simulink model "Commande"  (R2020b)
settings: Solver=VariableStepAuto  StartTime=0.0  StopTime=1  RelTol=1e-3
undefined symbols (not defined in the file or in its folder): FC, FuelCellLoadFcn, gcbh, ln, sps_rtmsupport, Ts
libraries: simulink x43, powerlib x37, powerlib_meascontrol x7, fuzblock x4, powerlib_extras x2
(part 2 of 3)

== system Commande/INC 1/Fuel Cell Stack/Model/Discrete//Detailed ==
  note: Break Algebraic
      | loop
  Current : Inport
  Op Temp : Inport  Port=2
  H2 : Inport  Port=3
  x_H2 : Inport  Port=4
  Air : Inport  Port=5
  y_O2 : Inport  Port=6
  Pf : Inport  Port=7
  PAir : Inport  Port=8
  Air consumption : Fcn  Expr=60000*FC.Nc*u(1)*FC.R*FC.Tstd/(4*FC.F*FC.Pstd*u(2))
  Bus Creator1 : BusCreator  Inputs=11
  CellVoltage : Subsystem
  Fcn2 : Fcn  Expr=u(1)-FC.Rohm*u(2)
  Fcn3 : Fcn  Expr=FC.Nc*u(1)/(FC.z*FC.F*u(2))*FC.Dh0
  Fuel consumption : Fcn  Expr=60000*FC.Nc*u(1)*FC.R*FC.Tstd/(FC.z*FC.F*FC.Pstd*u(2))
  Gain1 : Gain  Gain=100
  Gain3 : Gain  Gain=100
  Mux{,1,3..4,6} (5 alike) : Mux  Inputs=2
  Product : Product  RndMeth=Zero
  Product1 : Product  Inputs=*/  RndMeth=Zero
  Product2 : Product  RndMeth=Zero
  Saturation1 : Saturate  UpperLimit=0.9999  LowerLimit=0.0001
  Saturation2 : Saturate  UpperLimit=0.9999  LowerLimit=0.0001
  Saturation3 : Saturate  UpperLimit=inf  LowerLimit=1e-6
  Saturation4 : Saturate  UpperLimit=inf  LowerLimit=1e-3
  Saturation6 : Saturate  UpperLimit=inf  LowerLimit=0.001
  Saturation7 : Saturate  UpperLimit=inf  LowerLimit=0.001
  Saturation8 : Saturate  UpperLimit=inf  LowerLimit=200
  Selector : Selector  InputPortWidth=2  IndexOptions=Index vector (dialog)  Indices=[2]  OutputSizes=1
  Unit Delay : UnitDelay  SampleTime=Ts  HasFrameUpgradeWarning=on
  zero avoider : Saturate  UpperLimit=inf  LowerLimit=1e-6  LinearizeAsGain=off
  zero avoider2 : Saturate  UpperLimit=inf  LowerLimit=0  LinearizeAsGain=off
  Voltage : Outport  VectorParamsAs1DForOutWhenUnconnected=off
  m : Outport  Port=2  VectorParamsAs1DForOutWhenUnconnected=off
  wires:
  [E] -> Mux/1
  CellVoltage/7(E) -> [E], Voltage/1
  CellVoltage/5(En) -> Bus Creator1/10  "Nerst voltage En (V)"
  Saturation2/1 -> Mux6/2, CellVoltage/6(y)  "Oxidant composition"
  CellVoltage/4(i0) -> Bus Creator1/9  "Exchange current i0 (A)"
  Product2/1 -> Bus Creator1/6  "Stack consumption (lpm) [Air(Yellow); Fuel(Magenta)]"
  Gain3/1 -> Bus Creator1/3  "Stack Efficiency (%)"
  CellVoltage/1(Fr_AirFuel) -> Bus Creator1/5, Product2/1  "Flow Rate (lpm [Air(Yellow); Fuel(Magenta)]"
  Fuel consumption/1 -> Mux3/2
  Air consumption/1 -> Mux3/1
  Gain1/1 -> Bus Creator1/7  "Utilization (%) [O2(Yellow); H2(Magenta)]"
  Selector/1 -> Mux4/2
  Mux3/1 -> Bus Creator1/4  "Stack consumption (Standard lpm) [Air(Yellow); Fuel(Magenta)]"
  Saturation4/1 -> CellVoltage/5(Air)  "Air flow rate / utilization"
  Saturation3/1 -> CellVoltage/3(H2)  "Fuel flow rate / utilization"
  Bus Creator1/1 -> m/1
  Mux6/1 -> Air consumption/1
  Mux1/1 -> Fuel consumption/1
  CellVoltage/2(Uf_O2H2) -> Product2/2, Gain1/1, Selector/1
  Unit Delay/1 -> Mux6/1, Mux4/1, Mux/2, Bus Creator1/2, Product/2, Mux1/1, CellVoltage/1(i)  "Current"
  Saturation8/1 -> CellVoltage/2(T)  "Operating temperature"
  Saturation7/1 -> CellVoltage/8(PAir)  "Air supply pression"
  Saturation6/1 -> CellVoltage/7(Pf)  "Fuel supply pression"
  Saturation1/1 -> Mux1/2, CellVoltage/4(x)  "Fuel composition"
  Mux4/1 -> Fcn3/1
  PAir/1 -> Saturation7/1
  Pf/1 -> Saturation6/1
  zero avoider2/1 -> Product1/1
  CellVoltage/6(Eoc) -> Bus Creator1/11  "Open circuit voltage Eoc (V)"
  CellVoltage/3(A) -> Bus Creator1/8  "Slope of Tafel curve"
  Air/1 -> Saturation4/1
  Mux/1 -> Fcn2/1
  Fcn2/1 -> Bus Creator1/1, Product/1  "Voltage"
  H2/1 -> Saturation3/1
  x_H2/1 -> Saturation1/1
  y_O2/1 -> Saturation2/1
  Op Temp/1 -> Saturation8/1
  Product/1 -> zero avoider2/1
  Fcn3/1 -> zero avoider/1
  Current/1 -> Unit Delay/1
  Product1/1 -> Gain3/1
  zero avoider/1 -> Product1/2

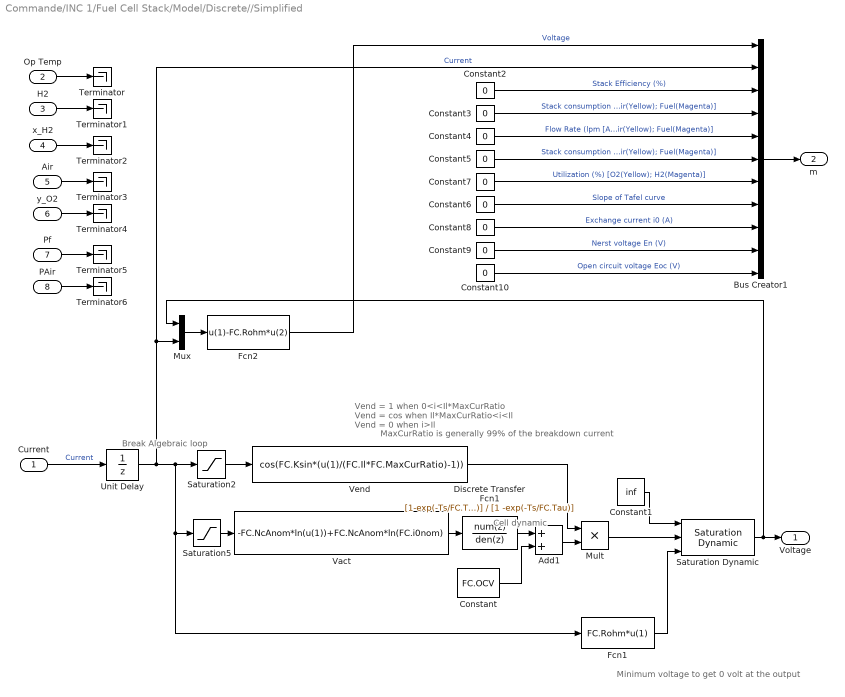
== system Commande/INC 1/Fuel Cell Stack/Model/Discrete//Simplified ==
  note: MaxCurRatio is generally 99% of the breakdown current
  note: Minimum voltage to get 0 volt at the output
  note: Cell dynamic
  note: Vend = 1 when 0<i<Il*MaxCurRatio
      | Vend = cos when Il*MaxCurRatio<i<Il
      | Vend = 0 when i>Il
  note: Break Algebraic
      | loop
  Current : Inport
  Op Temp : Inport  Port=2
  H2 : Inport  Port=3
  x_H2 : Inport  Port=4
  Air : Inport  Port=5
  y_O2 : Inport  Port=6
  Pf : Inport  Port=7
  PAir : Inport  Port=8
  Add1 : Sum
  Bus Creator1 : BusCreator  Inputs=11
  Constant : Constant  Value=FC.OCV
  Constant1 : Constant  Value=inf
  Constant{2..10} (9 alike) : Constant  Value=0
  Discrete Transfer Fcn1 : DiscreteTransferFcn  Numerator=[1-exp(-Ts/FC.Tau)]  Denominator=[1 -exp(-Ts/FC.Tau)]  SampleTime=Ts
  Fcn1 : Fcn  Expr=FC.Rohm*u(1)
  Fcn2 : Fcn  Expr=u(1)-FC.Rohm*u(2)
  Mult : Product
  Mux : Mux  Inputs=2
  Saturation Dynamic : simulink/Discontinuities/Saturation Dynamic  OutMin=[]  OutMax=[]  OutDataTypeStr=Inherit: Same as second input  OutDataType=fixdt(1, 16)  OutScaling=2^-10  DoSatur=off
  Saturation2 : Saturate  UpperLimit=FC.Il  LowerLimit=FC.Il*FC.MaxCurRatio  LinearizeAsGain=off
  Saturation5 : Saturate  UpperLimit=inf  LowerLimit=FC.i0nom  LinearizeAsGain=off
  Terminator{,1..6} (7 alike) : Terminator
  Unit Delay : UnitDelay  SampleTime=Ts  HasFrameUpgradeWarning=on
  Vact : Fcn  Expr=-FC.NcAnom*ln(u(1))+FC.NcAnom*ln(FC.i0nom)
  Vend : Fcn  Expr=cos(FC.Ksin*(u(1)/(FC.Il*FC.MaxCurRatio)-1))
  Voltage : Outport  VectorParamsAs1DForOutWhenUnconnected=off
  m : Outport  Port=2  VectorParamsAs1DForOutWhenUnconnected=off
  wires:
  Fcn2/1 -> Bus Creator1/1  "Voltage"
  Constant9/1 -> Bus Creator1/10  "Nerst voltage En (V)"
  Constant8/1 -> Bus Creator1/9  "Exchange current i0 (A)"
  Constant5/1 -> Bus Creator1/6  "Stack consumption (lpm) [Air(Yellow); Fuel(Magenta)]"
  Constant2/1 -> Bus Creator1/3  "Stack Efficiency (%)"
  Constant4/1 -> Bus Creator1/5  "Flow Rate (lpm [Air(Yellow); Fuel(Magenta)]"
  Constant7/1 -> Bus Creator1/7  "Utilization (%) [O2(Yellow); H2(Magenta)]"
  Constant3/1 -> Bus Creator1/4  "Stack consumption (Standard lpm) [Air(Yellow); Fuel(Magenta)]"
  Bus Creator1/1 -> m/1
  Constant10/1 -> Bus Creator1/11  "Open circuit voltage Eoc (V)"
  Constant6/1 -> Bus Creator1/8  "Slope of Tafel curve"
  PAir/1 -> Terminator6/1
  Pf/1 -> Terminator5/1
  Unit Delay/1 -> Bus Creator1/2, Mux/2, Fcn1/1, Saturation5/1, Saturation2/1  "Current"
  Saturation2/1 -> Vend/1
  Vend/1 -> Mult/1
  Mult/1 -> Saturation Dynamic/2
  Add1/1 -> Mult/2
  Vact/1 -> Discrete Transfer Fcn1/1
  Fcn1/1 -> Saturation Dynamic/3
  Constant1/1 -> Saturation Dynamic/1
  Constant/1 -> Add1/2
  Discrete Transfer Fcn1/1 -> Add1/1
  Saturation Dynamic/1 -> Mux/1, Voltage/1
  y_O2/1 -> Terminator4/1
  Air/1 -> Terminator3/1
  x_H2/1 -> Terminator2/1
  H2/1 -> Terminator1/1
  Op Temp/1 -> Terminator/1
  Current/1 -> Unit Delay/1  "Current"
  Saturation5/1 -> Vact/1
  Mux/1 -> Fcn2/1

== system Commande/P&O/Fuel Cell Stack/Model/Continuous//Detailed ==
  note: Break Algebraic
      | loop
  Current : Inport
  Op Temp : Inport  Port=2
  H2 : Inport  Port=3
  x_H2 : Inport  Port=4
  Air : Inport  Port=5
  y_O2 : Inport  Port=6
  Pf : Inport  Port=7
  PAir : Inport  Port=8
  Air consumption : Fcn  Expr=60000*FC.Nc*u(1)*FC.R*FC.Tstd/(4*FC.F*FC.Pstd*u(2))
  Bus Creator1 : BusCreator  Inputs=11
  CellVoltage : Subsystem
  Constant : Constant  Value=FC.Rohm
  Fcn2 : Fcn  Expr=u(1)-FC.Rohm*u(2)
  Fcn3 : Fcn  Expr=FC.Nc*u(1)/(FC.z*FC.F*u(2))*FC.Dh0
  Fuel consumption : Fcn  Expr=60000*FC.Nc*u(1)*FC.R*FC.Tstd/(FC.z*FC.F*FC.Pstd*u(2))
  Gain1 : Gain  Gain=100
  Gain3 : Gain  Gain=100
  Mux{,1,3..4,6} (5 alike) : Mux  Inputs=2
  Product : Product  RndMeth=Zero
  Product1 : Product  Inputs=*/  RndMeth=Zero
  Product2 : Product  RndMeth=Zero
  Saturation1 : Saturate  UpperLimit=0.9999  LowerLimit=0.0001
  Saturation2 : Saturate  UpperLimit=0.9999  LowerLimit=0.0001
  Saturation3 : Saturate  UpperLimit=inf  LowerLimit=1e-6
  Saturation4 : Saturate  UpperLimit=inf  LowerLimit=1e-3
  Saturation6 : Saturate  UpperLimit=inf  LowerLimit=0.001
  Saturation7 : Saturate  UpperLimit=inf  LowerLimit=0.001
  Saturation8 : Saturate  UpperLimit=inf  LowerLimit=200
  Selector : Selector  InputPortWidth=2  IndexOptions=Index vector (dialog)  Indices=[2]  OutputSizes=1
  Transfer Fcn : TransferFcn  Denominator=[1e-6 1]
  zero avoider : Saturate  UpperLimit=inf  LowerLimit=1e-6  LinearizeAsGain=off
  zero avoider2 : Saturate  UpperLimit=inf  LowerLimit=0  LinearizeAsGain=off
  Voltage : Outport  VectorParamsAs1DForOutWhenUnconnected=off
  m : Outport  Port=2  VectorParamsAs1DForOutWhenUnconnected=off
  wires:
  [E] -> Mux/1
  CellVoltage/7(E) -> Voltage/1, [E]
  CellVoltage/5(En) -> Bus Creator1/10  "Nerst voltage En (V)"
  Saturation2/1 -> Mux6/2, CellVoltage/6(y)  "Oxidant composition"
  CellVoltage/4(i0) -> Bus Creator1/9  "Exchange current i0 (A)"
  Product2/1 -> Bus Creator1/6  "Stack consumption (lpm) [Air(Yellow); Fuel(Magenta)]"
  Gain3/1 -> Bus Creator1/3  "Stack Efficiency (%)"
  CellVoltage/1(Fr_AirFuel) -> Bus Creator1/5, Product2/1  "Flow Rate (lpm [Air(Yellow); Fuel(Magenta)]"
  Fuel consumption/1 -> Mux3/2
  Air consumption/1 -> Mux3/1
  Gain1/1 -> Bus Creator1/7  "Utilization (%) [O2(Yellow); H2(Magenta)]"
  Selector/1 -> Mux4/2
  Mux3/1 -> Bus Creator1/4  "Stack consumption (Standard lpm) [Air(Yellow); Fuel(Magenta)]"
  Saturation4/1 -> CellVoltage/5(Air)  "Air flow rate / utilization"
  Saturation3/1 -> CellVoltage/3(H2)  "Fuel flow rate / utilization"
  Bus Creator1/1 -> m/1
  Mux6/1 -> Air consumption/1
  Mux1/1 -> Fuel consumption/1
  CellVoltage/2(Uf_O2H2) -> Product2/2, Gain1/1, Selector/1
  Transfer Fcn/1 -> Mux6/1, Mux4/1, Mux/2, Bus Creator1/2, Product/2, Mux1/1, CellVoltage/1(i)  "Current"
  Saturation8/1 -> CellVoltage/2(T)  "Operating temperature"
  Saturation7/1 -> CellVoltage/8(PAir)  "Air supply pression"
  Saturation6/1 -> CellVoltage/7(Pf)  "Fuel supply pression"
  Saturation1/1 -> Mux1/2, CellVoltage/4(x)  "Fuel composition"
  Mux4/1 -> Fcn3/1
  PAir/1 -> Saturation7/1
  Pf/1 -> Saturation6/1
  zero avoider2/1 -> Product1/1
  CellVoltage/6(Eoc) -> Bus Creator1/11  "Open circuit voltage Eoc (V)"
  CellVoltage/3(A) -> Bus Creator1/8  "Slope of Tafel curve"
  Air/1 -> Saturation4/1
  Mux/1 -> Fcn2/1
  Fcn2/1 -> Bus Creator1/1, Product/1  "Voltage"
  H2/1 -> Saturation3/1
  x_H2/1 -> Saturation1/1
  y_O2/1 -> Saturation2/1
  Op Temp/1 -> Saturation8/1
  Product/1 -> zero avoider2/1
  Fcn3/1 -> zero avoider/1
  Current/1 -> Transfer Fcn/1
  Product1/1 -> Gain3/1
  zero avoider/1 -> Product1/2

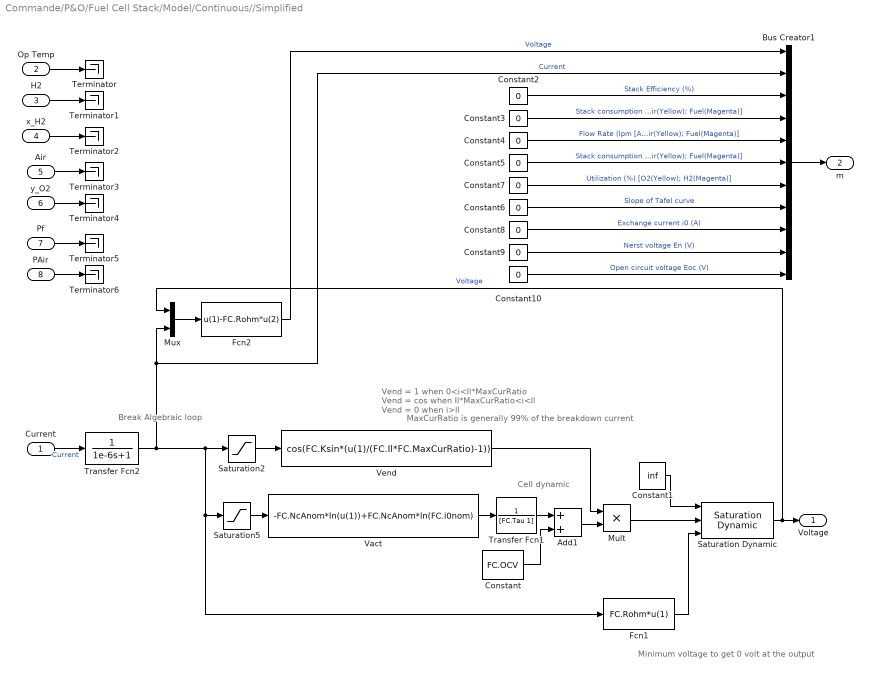
== system Commande/P&O/Fuel Cell Stack/Model/Continuous//Simplified ==
  note: MaxCurRatio is generally 99% of the breakdown current
  note: Minimum voltage to get 0 volt at the output
  note: Cell dynamic
  note: Vend = 1 when 0<i<Il*MaxCurRatio
      | Vend = cos when Il*MaxCurRatio<i<Il
      | Vend = 0 when i>Il
  note: Break Algebraic
      | loop
  Current : Inport
  Op Temp : Inport  Port=2
  H2 : Inport  Port=3
  x_H2 : Inport  Port=4
  Air : Inport  Port=5
  y_O2 : Inport  Port=6
  Pf : Inport  Port=7
  PAir : Inport  Port=8
  Add1 : Sum
  Bus Creator1 : BusCreator  Inputs=11
  Constant : Constant  Value=FC.OCV
  Constant1 : Constant  Value=inf
  Constant{2..10} (9 alike) : Constant  Value=0
  Fcn1 : Fcn  Expr=FC.Rohm*u(1)
  Fcn2 : Fcn  Expr=u(1)-FC.Rohm*u(2)
  Mult : Product
  Mux : Mux  Inputs=2
  Saturation Dynamic : simulink/Discontinuities/Saturation Dynamic  OutMin=[]  OutMax=[]  OutDataTypeStr=Inherit: Same as second input  OutDataType=fixdt(1, 16)  OutScaling=2^-10  DoSatur=off
  Saturation2 : Saturate  UpperLimit=FC.Il  LowerLimit=FC.Il*FC.MaxCurRatio  LinearizeAsGain=off
  Saturation5 : Saturate  UpperLimit=inf  LowerLimit=FC.i0nom  LinearizeAsGain=off
  Terminator{,1..6} (7 alike) : Terminator
  Transfer Fcn1 : TransferFcn  Denominator=[FC.Tau 1]
  Transfer Fcn2 : TransferFcn  Denominator=[1e-6 1]
  Vact : Fcn  Expr=-FC.NcAnom*ln(u(1))+FC.NcAnom*ln(FC.i0nom)
  Vend : Fcn  Expr=cos(FC.Ksin*(u(1)/(FC.Il*FC.MaxCurRatio)-1))
  Voltage : Outport  VectorParamsAs1DForOutWhenUnconnected=off
  m : Outport  Port=2  VectorParamsAs1DForOutWhenUnconnected=off
  wires:
  Constant9/1 -> Bus Creator1/10  "Nerst voltage En (V)"
  Constant8/1 -> Bus Creator1/9  "Exchange current i0 (A)"
  Constant5/1 -> Bus Creator1/6  "Stack consumption (lpm) [Air(Yellow); Fuel(Magenta)]"
  Constant2/1 -> Bus Creator1/3  "Stack Efficiency (%)"
  Constant4/1 -> Bus Creator1/5  "Flow Rate (lpm [Air(Yellow); Fuel(Magenta)]"
  Constant7/1 -> Bus Creator1/7  "Utilization (%) [O2(Yellow); H2(Magenta)]"
  Constant3/1 -> Bus Creator1/4  "Stack consumption (Standard lpm) [Air(Yellow); Fuel(Magenta)]"
  Bus Creator1/1 -> m/1
  Constant10/1 -> Bus Creator1/11  "Open circuit voltage Eoc (V)"
  Constant6/1 -> Bus Creator1/8  "Slope of Tafel curve"
  Fcn2/1 -> Bus Creator1/1  "Voltage"
  PAir/1 -> Terminator6/1
  Pf/1 -> Terminator5/1
  Transfer Fcn2/1 -> Bus Creator1/2, Mux/2, Fcn1/1, Saturation5/1, Saturation2/1  "Current"
  Saturation2/1 -> Vend/1
  Vend/1 -> Mult/1
  Mult/1 -> Saturation Dynamic/2
  Add1/1 -> Mult/2
  Vact/1 -> Transfer Fcn1/1
  Fcn1/1 -> Saturation Dynamic/3
  Constant1/1 -> Saturation Dynamic/1
  Constant/1 -> Add1/2
  Transfer Fcn1/1 -> Add1/1
  Saturation Dynamic/1 -> Mux/1, Voltage/1  "Voltage"
  y_O2/1 -> Terminator4/1
  Air/1 -> Terminator3/1
  x_H2/1 -> Terminator2/1
  H2/1 -> Terminator1/1
  Op Temp/1 -> Terminator/1
  Current/1 -> Transfer Fcn2/1  "Current"
  Saturation5/1 -> Vact/1
  Mux/1 -> Fcn2/1

== system Commande/P&O/Fuel Cell Stack/Model/Discrete//Detailed ==
  note: Break Algebraic
      | loop
  Current : Inport
  Op Temp : Inport  Port=2
  H2 : Inport  Port=3
  x_H2 : Inport  Port=4
  Air : Inport  Port=5
  y_O2 : Inport  Port=6
  Pf : Inport  Port=7
  PAir : Inport  Port=8
  Air consumption : Fcn  Expr=60000*FC.Nc*u(1)*FC.R*FC.Tstd/(4*FC.F*FC.Pstd*u(2))
  Bus Creator1 : BusCreator  Inputs=11
  CellVoltage : Subsystem
  Fcn2 : Fcn  Expr=u(1)-FC.Rohm*u(2)
  Fcn3 : Fcn  Expr=FC.Nc*u(1)/(FC.z*FC.F*u(2))*FC.Dh0
  Fuel consumption : Fcn  Expr=60000*FC.Nc*u(1)*FC.R*FC.Tstd/(FC.z*FC.F*FC.Pstd*u(2))
  Gain1 : Gain  Gain=100
  Gain3 : Gain  Gain=100
  Mux{,1,3..4,6} (5 alike) : Mux  Inputs=2
  Product : Product  RndMeth=Zero
  Product1 : Product  Inputs=*/  RndMeth=Zero
  Product2 : Product  RndMeth=Zero
  Saturation1 : Saturate  UpperLimit=0.9999  LowerLimit=0.0001
  Saturation2 : Saturate  UpperLimit=0.9999  LowerLimit=0.0001
  Saturation3 : Saturate  UpperLimit=inf  LowerLimit=1e-6
  Saturation4 : Saturate  UpperLimit=inf  LowerLimit=1e-3
  Saturation6 : Saturate  UpperLimit=inf  LowerLimit=0.001
  Saturation7 : Saturate  UpperLimit=inf  LowerLimit=0.001
  Saturation8 : Saturate  UpperLimit=inf  LowerLimit=200
  Selector : Selector  InputPortWidth=2  IndexOptions=Index vector (dialog)  Indices=[2]  OutputSizes=1
  Unit Delay : UnitDelay  SampleTime=Ts  HasFrameUpgradeWarning=on
  zero avoider : Saturate  UpperLimit=inf  LowerLimit=1e-6  LinearizeAsGain=off
  zero avoider2 : Saturate  UpperLimit=inf  LowerLimit=0  LinearizeAsGain=off
  Voltage : Outport  VectorParamsAs1DForOutWhenUnconnected=off
  m : Outport  Port=2  VectorParamsAs1DForOutWhenUnconnected=off
  wires:
  [E] -> Mux/1
  CellVoltage/7(E) -> [E], Voltage/1
  CellVoltage/5(En) -> Bus Creator1/10  "Nerst voltage En (V)"
  Saturation2/1 -> Mux6/2, CellVoltage/6(y)  "Oxidant composition"
  CellVoltage/4(i0) -> Bus Creator1/9  "Exchange current i0 (A)"
  Product2/1 -> Bus Creator1/6  "Stack consumption (lpm) [Air(Yellow); Fuel(Magenta)]"
  Gain3/1 -> Bus Creator1/3  "Stack Efficiency (%)"
  CellVoltage/1(Fr_AirFuel) -> Bus Creator1/5, Product2/1  "Flow Rate (lpm [Air(Yellow); Fuel(Magenta)]"
  Fuel consumption/1 -> Mux3/2
  Air consumption/1 -> Mux3/1
  Gain1/1 -> Bus Creator1/7  "Utilization (%) [O2(Yellow); H2(Magenta)]"
  Selector/1 -> Mux4/2
  Mux3/1 -> Bus Creator1/4  "Stack consumption (Standard lpm) [Air(Yellow); Fuel(Magenta)]"
  Saturation4/1 -> CellVoltage/5(Air)  "Air flow rate / utilization"
  Saturation3/1 -> CellVoltage/3(H2)  "Fuel flow rate / utilization"
  Bus Creator1/1 -> m/1
  Mux6/1 -> Air consumption/1
  Mux1/1 -> Fuel consumption/1
  CellVoltage/2(Uf_O2H2) -> Product2/2, Gain1/1, Selector/1
  Unit Delay/1 -> Mux6/1, Mux4/1, Mux/2, Bus Creator1/2, Product/2, Mux1/1, CellVoltage/1(i)  "Current"
  Saturation8/1 -> CellVoltage/2(T)  "Operating temperature"
  Saturation7/1 -> CellVoltage/8(PAir)  "Air supply pression"
  Saturation6/1 -> CellVoltage/7(Pf)  "Fuel supply pression"
  Saturation1/1 -> Mux1/2, CellVoltage/4(x)  "Fuel composition"
  Mux4/1 -> Fcn3/1
  PAir/1 -> Saturation7/1
  Pf/1 -> Saturation6/1
  zero avoider2/1 -> Product1/1
  CellVoltage/6(Eoc) -> Bus Creator1/11  "Open circuit voltage Eoc (V)"
  CellVoltage/3(A) -> Bus Creator1/8  "Slope of Tafel curve"
  Air/1 -> Saturation4/1
  Mux/1 -> Fcn2/1
  Fcn2/1 -> Bus Creator1/1, Product/1  "Voltage"
  H2/1 -> Saturation3/1
  x_H2/1 -> Saturation1/1
  y_O2/1 -> Saturation2/1
  Op Temp/1 -> Saturation8/1
  Product/1 -> zero avoider2/1
  Fcn3/1 -> zero avoider/1
  Current/1 -> Unit Delay/1
  Product1/1 -> Gain3/1
  zero avoider/1 -> Product1/2

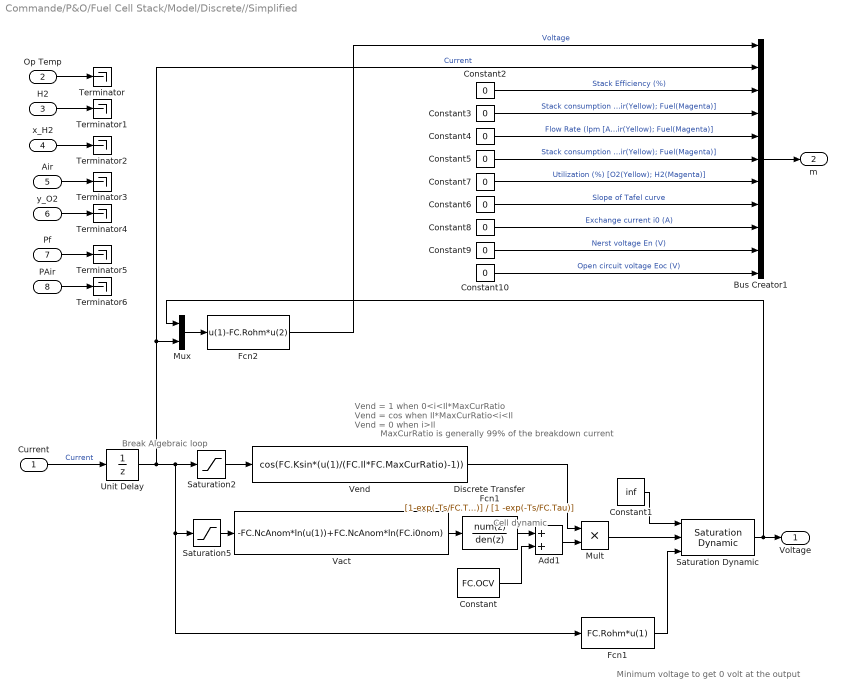
== system Commande/P&O/Fuel Cell Stack/Model/Discrete//Simplified ==
  note: MaxCurRatio is generally 99% of the breakdown current
  note: Minimum voltage to get 0 volt at the output
  note: Cell dynamic
  note: Vend = 1 when 0<i<Il*MaxCurRatio
      | Vend = cos when Il*MaxCurRatio<i<Il
      | Vend = 0 when i>Il
  note: Break Algebraic
      | loop
  Current : Inport
  Op Temp : Inport  Port=2
  H2 : Inport  Port=3
  x_H2 : Inport  Port=4
  Air : Inport  Port=5
  y_O2 : Inport  Port=6
  Pf : Inport  Port=7
  PAir : Inport  Port=8
  Add1 : Sum
  Bus Creator1 : BusCreator  Inputs=11
  Constant : Constant  Value=FC.OCV
  Constant1 : Constant  Value=inf
  Constant{2..10} (9 alike) : Constant  Value=0
  Discrete Transfer Fcn1 : DiscreteTransferFcn  Numerator=[1-exp(-Ts/FC.Tau)]  Denominator=[1 -exp(-Ts/FC.Tau)]  SampleTime=Ts
  Fcn1 : Fcn  Expr=FC.Rohm*u(1)
  Fcn2 : Fcn  Expr=u(1)-FC.Rohm*u(2)
  Mult : Product
  Mux : Mux  Inputs=2
  Saturation Dynamic : simulink/Discontinuities/Saturation Dynamic  OutMin=[]  OutMax=[]  OutDataTypeStr=Inherit: Same as second input  OutDataType=fixdt(1, 16)  OutScaling=2^-10  DoSatur=off
  Saturation2 : Saturate  UpperLimit=FC.Il  LowerLimit=FC.Il*FC.MaxCurRatio  LinearizeAsGain=off
  Saturation5 : Saturate  UpperLimit=inf  LowerLimit=FC.i0nom  LinearizeAsGain=off
  Terminator{,1..6} (7 alike) : Terminator
  Unit Delay : UnitDelay  SampleTime=Ts  HasFrameUpgradeWarning=on
  Vact : Fcn  Expr=-FC.NcAnom*ln(u(1))+FC.NcAnom*ln(FC.i0nom)
  Vend : Fcn  Expr=cos(FC.Ksin*(u(1)/(FC.Il*FC.MaxCurRatio)-1))
  Voltage : Outport  VectorParamsAs1DForOutWhenUnconnected=off
  m : Outport  Port=2  VectorParamsAs1DForOutWhenUnconnected=off
  wires:
  Fcn2/1 -> Bus Creator1/1  "Voltage"
  Constant9/1 -> Bus Creator1/10  "Nerst voltage En (V)"
  Constant8/1 -> Bus Creator1/9  "Exchange current i0 (A)"
  Constant5/1 -> Bus Creator1/6  "Stack consumption (lpm) [Air(Yellow); Fuel(Magenta)]"
  Constant2/1 -> Bus Creator1/3  "Stack Efficiency (%)"
  Constant4/1 -> Bus Creator1/5  "Flow Rate (lpm [Air(Yellow); Fuel(Magenta)]"
  Constant7/1 -> Bus Creator1/7  "Utilization (%) [O2(Yellow); H2(Magenta)]"
  Constant3/1 -> Bus Creator1/4  "Stack consumption (Standard lpm) [Air(Yellow); Fuel(Magenta)]"
  Bus Creator1/1 -> m/1
  Constant10/1 -> Bus Creator1/11  "Open circuit voltage Eoc (V)"
  Constant6/1 -> Bus Creator1/8  "Slope of Tafel curve"
  PAir/1 -> Terminator6/1
  Pf/1 -> Terminator5/1
  Unit Delay/1 -> Bus Creator1/2, Mux/2, Fcn1/1, Saturation5/1, Saturation2/1  "Current"
  Saturation2/1 -> Vend/1
  Vend/1 -> Mult/1
  Mult/1 -> Saturation Dynamic/2
  Add1/1 -> Mult/2
  Vact/1 -> Discrete Transfer Fcn1/1
  Fcn1/1 -> Saturation Dynamic/3
  Constant1/1 -> Saturation Dynamic/1
  Constant/1 -> Add1/2
  Discrete Transfer Fcn1/1 -> Add1/1
  Saturation Dynamic/1 -> Mux/1, Voltage/1
  y_O2/1 -> Terminator4/1
  Air/1 -> Terminator3/1
  x_H2/1 -> Terminator2/1
  H2/1 -> Terminator1/1
  Op Temp/1 -> Terminator/1
  Current/1 -> Unit Delay/1  "Current"
  Saturation5/1 -> Vact/1
  Mux/1 -> Fcn2/1

== system Commande/fuzzy logic/Fuel Cell Stack1/Model/Continuous//Detailed ==
  note: Break Algebraic
      | loop
  Current : Inport
  Op Temp : Inport  Port=2
  H2 : Inport  Port=3
  x_H2 : Inport  Port=4
  Air : Inport  Port=5
  y_O2 : Inport  Port=6
  Pf : Inport  Port=7
  PAir : Inport  Port=8
  Air consumption : Fcn  Expr=60000*FC.Nc*u(1)*FC.R*FC.Tstd/(4*FC.F*FC.Pstd*u(2))
  Bus Creator1 : BusCreator  Inputs=11
  CellVoltage : Subsystem
  Constant : Constant  Value=FC.Rohm
  Fcn2 : Fcn  Expr=u(1)-FC.Rohm*u(2)
  Fcn3 : Fcn  Expr=FC.Nc*u(1)/(FC.z*FC.F*u(2))*FC.Dh0
  Fuel consumption : Fcn  Expr=60000*FC.Nc*u(1)*FC.R*FC.Tstd/(FC.z*FC.F*FC.Pstd*u(2))
  Gain1 : Gain  Gain=100
  Gain3 : Gain  Gain=100
  Mux{,1,3..4,6} (5 alike) : Mux  Inputs=2
  Product : Product  RndMeth=Zero
  Product1 : Product  Inputs=*/  RndMeth=Zero
  Product2 : Product  RndMeth=Zero
  Saturation1 : Saturate  UpperLimit=0.9999  LowerLimit=0.0001
  Saturation2 : Saturate  UpperLimit=0.9999  LowerLimit=0.0001
  Saturation3 : Saturate  UpperLimit=inf  LowerLimit=1e-6
  Saturation4 : Saturate  UpperLimit=inf  LowerLimit=1e-3
  Saturation6 : Saturate  UpperLimit=inf  LowerLimit=0.001
  Saturation7 : Saturate  UpperLimit=inf  LowerLimit=0.001
  Saturation8 : Saturate  UpperLimit=inf  LowerLimit=200
  Selector : Selector  InputPortWidth=2  IndexOptions=Index vector (dialog)  Indices=[2]  OutputSizes=1
  Transfer Fcn : TransferFcn  Denominator=[1e-6 1]
  zero avoider : Saturate  UpperLimit=inf  LowerLimit=1e-6  LinearizeAsGain=off
  zero avoider2 : Saturate  UpperLimit=inf  LowerLimit=0  LinearizeAsGain=off
  Voltage : Outport  VectorParamsAs1DForOutWhenUnconnected=off
  m : Outport  Port=2  VectorParamsAs1DForOutWhenUnconnected=off
  wires:
  [E] -> Mux/1
  CellVoltage/7(E) -> Voltage/1, [E]
  CellVoltage/5(En) -> Bus Creator1/10  "Nerst voltage En (V)"
  Saturation2/1 -> Mux6/2, CellVoltage/6(y)  "Oxidant composition"
  CellVoltage/4(i0) -> Bus Creator1/9  "Exchange current i0 (A)"
  Product2/1 -> Bus Creator1/6  "Stack consumption (lpm) [Air(Yellow); Fuel(Magenta)]"
  Gain3/1 -> Bus Creator1/3  "Stack Efficiency (%)"
  CellVoltage/1(Fr_AirFuel) -> Bus Creator1/5, Product2/1  "Flow Rate (lpm [Air(Yellow); Fuel(Magenta)]"
  Fuel consumption/1 -> Mux3/2
  Air consumption/1 -> Mux3/1
  Gain1/1 -> Bus Creator1/7  "Utilization (%) [O2(Yellow); H2(Magenta)]"
  Selector/1 -> Mux4/2
  Mux3/1 -> Bus Creator1/4  "Stack consumption (Standard lpm) [Air(Yellow); Fuel(Magenta)]"
  Saturation4/1 -> CellVoltage/5(Air)  "Air flow rate / utilization"
  Saturation3/1 -> CellVoltage/3(H2)  "Fuel flow rate / utilization"
  Bus Creator1/1 -> m/1
  Mux6/1 -> Air consumption/1
  Mux1/1 -> Fuel consumption/1
  CellVoltage/2(Uf_O2H2) -> Product2/2, Gain1/1, Selector/1
  Transfer Fcn/1 -> Mux6/1, Mux4/1, Mux/2, Bus Creator1/2, Product/2, Mux1/1, CellVoltage/1(i)  "Current"
  Saturation8/1 -> CellVoltage/2(T)  "Operating temperature"
  Saturation7/1 -> CellVoltage/8(PAir)  "Air supply pression"
  Saturation6/1 -> CellVoltage/7(Pf)  "Fuel supply pression"
  Saturation1/1 -> Mux1/2, CellVoltage/4(x)  "Fuel composition"
  Mux4/1 -> Fcn3/1
  PAir/1 -> Saturation7/1
  Pf/1 -> Saturation6/1
  zero avoider2/1 -> Product1/1
  CellVoltage/6(Eoc) -> Bus Creator1/11  "Open circuit voltage Eoc (V)"
  CellVoltage/3(A) -> Bus Creator1/8  "Slope of Tafel curve"
  Air/1 -> Saturation4/1
  Mux/1 -> Fcn2/1
  Fcn2/1 -> Bus Creator1/1, Product/1  "Voltage"
  H2/1 -> Saturation3/1
  x_H2/1 -> Saturation1/1
  y_O2/1 -> Saturation2/1
  Op Temp/1 -> Saturation8/1
  Product/1 -> zero avoider2/1
  Fcn3/1 -> zero avoider/1
  Current/1 -> Transfer Fcn/1
  Product1/1 -> Gain3/1
  zero avoider/1 -> Product1/2

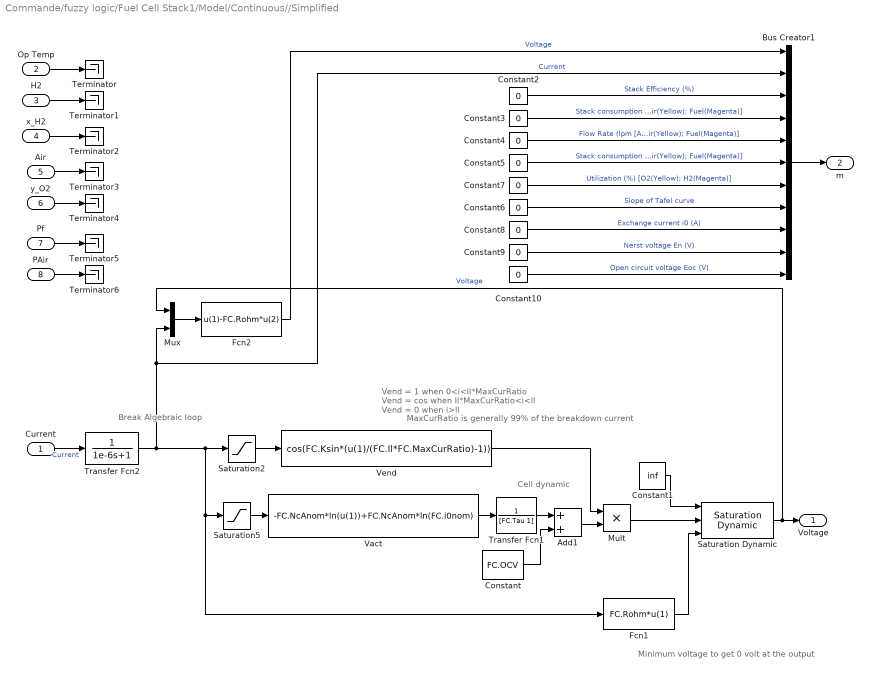
== system Commande/fuzzy logic/Fuel Cell Stack1/Model/Continuous//Simplified ==
  note: MaxCurRatio is generally 99% of the breakdown current
  note: Minimum voltage to get 0 volt at the output
  note: Cell dynamic
  note: Vend = 1 when 0<i<Il*MaxCurRatio
      | Vend = cos when Il*MaxCurRatio<i<Il
      | Vend = 0 when i>Il
  note: Break Algebraic
      | loop
  Current : Inport
  Op Temp : Inport  Port=2
  H2 : Inport  Port=3
  x_H2 : Inport  Port=4
  Air : Inport  Port=5
  y_O2 : Inport  Port=6
  Pf : Inport  Port=7
  PAir : Inport  Port=8
  Add1 : Sum
  Bus Creator1 : BusCreator  Inputs=11
  Constant : Constant  Value=FC.OCV
  Constant1 : Constant  Value=inf
  Constant{2..10} (9 alike) : Constant  Value=0
  Fcn1 : Fcn  Expr=FC.Rohm*u(1)
  Fcn2 : Fcn  Expr=u(1)-FC.Rohm*u(2)
  Mult : Product
  Mux : Mux  Inputs=2
  Saturation Dynamic : simulink/Discontinuities/Saturation Dynamic  OutMin=[]  OutMax=[]  OutDataTypeStr=Inherit: Same as second input  OutDataType=fixdt(1, 16)  OutScaling=2^-10  DoSatur=off
  Saturation2 : Saturate  UpperLimit=FC.Il  LowerLimit=FC.Il*FC.MaxCurRatio  LinearizeAsGain=off
  Saturation5 : Saturate  UpperLimit=inf  LowerLimit=FC.i0nom  LinearizeAsGain=off
  Terminator{,1..6} (7 alike) : Terminator
  Transfer Fcn1 : TransferFcn  Denominator=[FC.Tau 1]
  Transfer Fcn2 : TransferFcn  Denominator=[1e-6 1]
  Vact : Fcn  Expr=-FC.NcAnom*ln(u(1))+FC.NcAnom*ln(FC.i0nom)
  Vend : Fcn  Expr=cos(FC.Ksin*(u(1)/(FC.Il*FC.MaxCurRatio)-1))
  Voltage : Outport  VectorParamsAs1DForOutWhenUnconnected=off
  m : Outport  Port=2  VectorParamsAs1DForOutWhenUnconnected=off
  wires:
  Constant9/1 -> Bus Creator1/10  "Nerst voltage En (V)"
  Constant8/1 -> Bus Creator1/9  "Exchange current i0 (A)"
  Constant5/1 -> Bus Creator1/6  "Stack consumption (lpm) [Air(Yellow); Fuel(Magenta)]"
  Constant2/1 -> Bus Creator1/3  "Stack Efficiency (%)"
  Constant4/1 -> Bus Creator1/5  "Flow Rate (lpm [Air(Yellow); Fuel(Magenta)]"
  Constant7/1 -> Bus Creator1/7  "Utilization (%) [O2(Yellow); H2(Magenta)]"
  Constant3/1 -> Bus Creator1/4  "Stack consumption (Standard lpm) [Air(Yellow); Fuel(Magenta)]"
  Bus Creator1/1 -> m/1
  Constant10/1 -> Bus Creator1/11  "Open circuit voltage Eoc (V)"
  Constant6/1 -> Bus Creator1/8  "Slope of Tafel curve"
  Fcn2/1 -> Bus Creator1/1  "Voltage"
  PAir/1 -> Terminator6/1
  Pf/1 -> Terminator5/1
  Transfer Fcn2/1 -> Bus Creator1/2, Mux/2, Fcn1/1, Saturation5/1, Saturation2/1  "Current"
  Saturation2/1 -> Vend/1
  Vend/1 -> Mult/1
  Mult/1 -> Saturation Dynamic/2
  Add1/1 -> Mult/2
  Vact/1 -> Transfer Fcn1/1
  Fcn1/1 -> Saturation Dynamic/3
  Constant1/1 -> Saturation Dynamic/1
  Constant/1 -> Add1/2
  Transfer Fcn1/1 -> Add1/1
  Saturation Dynamic/1 -> Mux/1, Voltage/1  "Voltage"
  y_O2/1 -> Terminator4/1
  Air/1 -> Terminator3/1
  x_H2/1 -> Terminator2/1
  H2/1 -> Terminator1/1
  Op Temp/1 -> Terminator/1
  Current/1 -> Transfer Fcn2/1  "Current"
  Saturation5/1 -> Vact/1
  Mux/1 -> Fcn2/1

== system Commande/fuzzy logic/Fuel Cell Stack1/Model/Discrete//Detailed ==
  note: Break Algebraic
      | loop
  Current : Inport
  Op Temp : Inport  Port=2
  H2 : Inport  Port=3
  x_H2 : Inport  Port=4
  Air : Inport  Port=5
  y_O2 : Inport  Port=6
  Pf : Inport  Port=7
  PAir : Inport  Port=8
  Air consumption : Fcn  Expr=60000*FC.Nc*u(1)*FC.R*FC.Tstd/(4*FC.F*FC.Pstd*u(2))
  Bus Creator1 : BusCreator  Inputs=11
  CellVoltage : Subsystem
  Fcn2 : Fcn  Expr=u(1)-FC.Rohm*u(2)
  Fcn3 : Fcn  Expr=FC.Nc*u(1)/(FC.z*FC.F*u(2))*FC.Dh0
  Fuel consumption : Fcn  Expr=60000*FC.Nc*u(1)*FC.R*FC.Tstd/(FC.z*FC.F*FC.Pstd*u(2))
  Gain1 : Gain  Gain=100
  Gain3 : Gain  Gain=100
  Mux{,1,3..4,6} (5 alike) : Mux  Inputs=2
  Product : Product  RndMeth=Zero
  Product1 : Product  Inputs=*/  RndMeth=Zero
  Product2 : Product  RndMeth=Zero
  Saturation1 : Saturate  UpperLimit=0.9999  LowerLimit=0.0001
  Saturation2 : Saturate  UpperLimit=0.9999  LowerLimit=0.0001
  Saturation3 : Saturate  UpperLimit=inf  LowerLimit=1e-6
  Saturation4 : Saturate  UpperLimit=inf  LowerLimit=1e-3
  Saturation6 : Saturate  UpperLimit=inf  LowerLimit=0.001
  Saturation7 : Saturate  UpperLimit=inf  LowerLimit=0.001
  Saturation8 : Saturate  UpperLimit=inf  LowerLimit=200
  Selector : Selector  InputPortWidth=2  IndexOptions=Index vector (dialog)  Indices=[2]  OutputSizes=1
  Unit Delay : UnitDelay  SampleTime=Ts  HasFrameUpgradeWarning=on
  zero avoider : Saturate  UpperLimit=inf  LowerLimit=1e-6  LinearizeAsGain=off
  zero avoider2 : Saturate  UpperLimit=inf  LowerLimit=0  LinearizeAsGain=off
  Voltage : Outport  VectorParamsAs1DForOutWhenUnconnected=off
  m : Outport  Port=2  VectorParamsAs1DForOutWhenUnconnected=off
  wires:
  [E] -> Mux/1
  CellVoltage/7(E) -> [E], Voltage/1
  CellVoltage/5(En) -> Bus Creator1/10  "Nerst voltage En (V)"
  Saturation2/1 -> Mux6/2, CellVoltage/6(y)  "Oxidant composition"
  CellVoltage/4(i0) -> Bus Creator1/9  "Exchange current i0 (A)"
  Product2/1 -> Bus Creator1/6  "Stack consumption (lpm) [Air(Yellow); Fuel(Magenta)]"
  Gain3/1 -> Bus Creator1/3  "Stack Efficiency (%)"
  CellVoltage/1(Fr_AirFuel) -> Bus Creator1/5, Product2/1  "Flow Rate (lpm [Air(Yellow); Fuel(Magenta)]"
  Fuel consumption/1 -> Mux3/2
  Air consumption/1 -> Mux3/1
  Gain1/1 -> Bus Creator1/7  "Utilization (%) [O2(Yellow); H2(Magenta)]"
  Selector/1 -> Mux4/2
  Mux3/1 -> Bus Creator1/4  "Stack consumption (Standard lpm) [Air(Yellow); Fuel(Magenta)]"
  Saturation4/1 -> CellVoltage/5(Air)  "Air flow rate / utilization"
  Saturation3/1 -> CellVoltage/3(H2)  "Fuel flow rate / utilization"
  Bus Creator1/1 -> m/1
  Mux6/1 -> Air consumption/1
  Mux1/1 -> Fuel consumption/1
  CellVoltage/2(Uf_O2H2) -> Product2/2, Gain1/1, Selector/1
  Unit Delay/1 -> Mux6/1, Mux4/1, Mux/2, Bus Creator1/2, Product/2, Mux1/1, CellVoltage/1(i)  "Current"
  Saturation8/1 -> CellVoltage/2(T)  "Operating temperature"
  Saturation7/1 -> CellVoltage/8(PAir)  "Air supply pression"
  Saturation6/1 -> CellVoltage/7(Pf)  "Fuel supply pression"
  Saturation1/1 -> Mux1/2, CellVoltage/4(x)  "Fuel composition"
  Mux4/1 -> Fcn3/1
  PAir/1 -> Saturation7/1
  Pf/1 -> Saturation6/1
  zero avoider2/1 -> Product1/1
  CellVoltage/6(Eoc) -> Bus Creator1/11  "Open circuit voltage Eoc (V)"
  CellVoltage/3(A) -> Bus Creator1/8  "Slope of Tafel curve"
  Air/1 -> Saturation4/1
  Mux/1 -> Fcn2/1
  Fcn2/1 -> Bus Creator1/1, Product/1  "Voltage"
  H2/1 -> Saturation3/1
  x_H2/1 -> Saturation1/1
  y_O2/1 -> Saturation2/1
  Op Temp/1 -> Saturation8/1
  Product/1 -> zero avoider2/1
  Fcn3/1 -> zero avoider/1
  Current/1 -> Unit Delay/1
  Product1/1 -> Gain3/1
  zero avoider/1 -> Product1/2

== system Commande/fuzzy logic/Fuel Cell Stack1/Model/Discrete//Simplified ==
  note: MaxCurRatio is generally 99% of the breakdown current
  note: Minimum voltage to get 0 volt at the output
  note: Cell dynamic
  note: Vend = 1 when 0<i<Il*MaxCurRatio
      | Vend = cos when Il*MaxCurRatio<i<Il
      | Vend = 0 when i>Il
  note: Break Algebraic
      | loop
  Current : Inport
  Op Temp : Inport  Port=2
  H2 : Inport  Port=3
  x_H2 : Inport  Port=4
  Air : Inport  Port=5
  y_O2 : Inport  Port=6
  Pf : Inport  Port=7
  PAir : Inport  Port=8
  Add1 : Sum
  Bus Creator1 : BusCreator  Inputs=11
  Constant : Constant  Value=FC.OCV
  Constant1 : Constant  Value=inf
  Constant{2..10} (9 alike) : Constant  Value=0
  Discrete Transfer Fcn1 : DiscreteTransferFcn  Numerator=[1-exp(-Ts/FC.Tau)]  Denominator=[1 -exp(-Ts/FC.Tau)]  SampleTime=Ts
  Fcn1 : Fcn  Expr=FC.Rohm*u(1)
  Fcn2 : Fcn  Expr=u(1)-FC.Rohm*u(2)
  Mult : Product
  Mux : Mux  Inputs=2
  Saturation Dynamic : simulink/Discontinuities/Saturation Dynamic  OutMin=[]  OutMax=[]  OutDataTypeStr=Inherit: Same as second input  OutDataType=fixdt(1, 16)  OutScaling=2^-10  DoSatur=off
  Saturation2 : Saturate  UpperLimit=FC.Il  LowerLimit=FC.Il*FC.MaxCurRatio  LinearizeAsGain=off
  Saturation5 : Saturate  UpperLimit=inf  LowerLimit=FC.i0nom  LinearizeAsGain=off
  Terminator{,1..6} (7 alike) : Terminator
  Unit Delay : UnitDelay  SampleTime=Ts  HasFrameUpgradeWarning=on
  Vact : Fcn  Expr=-FC.NcAnom*ln(u(1))+FC.NcAnom*ln(FC.i0nom)
  Vend : Fcn  Expr=cos(FC.Ksin*(u(1)/(FC.Il*FC.MaxCurRatio)-1))
  Voltage : Outport  VectorParamsAs1DForOutWhenUnconnected=off
  m : Outport  Port=2  VectorParamsAs1DForOutWhenUnconnected=off
  wires:
  Fcn2/1 -> Bus Creator1/1  "Voltage"
  Constant9/1 -> Bus Creator1/10  "Nerst voltage En (V)"
  Constant8/1 -> Bus Creator1/9  "Exchange current i0 (A)"
  Constant5/1 -> Bus Creator1/6  "Stack consumption (lpm) [Air(Yellow); Fuel(Magenta)]"
  Constant2/1 -> Bus Creator1/3  "Stack Efficiency (%)"
  Constant4/1 -> Bus Creator1/5  "Flow Rate (lpm [Air(Yellow); Fuel(Magenta)]"
  Constant7/1 -> Bus Creator1/7  "Utilization (%) [O2(Yellow); H2(Magenta)]"
  Constant3/1 -> Bus Creator1/4  "Stack consumption (Standard lpm) [Air(Yellow); Fuel(Magenta)]"
  Bus Creator1/1 -> m/1
  Constant10/1 -> Bus Creator1/11  "Open circuit voltage Eoc (V)"
  Constant6/1 -> Bus Creator1/8  "Slope of Tafel curve"
  PAir/1 -> Terminator6/1
  Pf/1 -> Terminator5/1
  Unit Delay/1 -> Bus Creator1/2, Mux/2, Fcn1/1, Saturation5/1, Saturation2/1  "Current"
  Saturation2/1 -> Vend/1
  Vend/1 -> Mult/1
  Mult/1 -> Saturation Dynamic/2
  Add1/1 -> Mult/2
  Vact/1 -> Discrete Transfer Fcn1/1
  Fcn1/1 -> Saturation Dynamic/3
  Constant1/1 -> Saturation Dynamic/1
  Constant/1 -> Add1/2
  Discrete Transfer Fcn1/1 -> Add1/1
  Saturation Dynamic/1 -> Mux/1, Voltage/1
  y_O2/1 -> Terminator4/1
  Air/1 -> Terminator3/1
  x_H2/1 -> Terminator2/1
  H2/1 -> Terminator1/1
  Op Temp/1 -> Terminator/1
  Current/1 -> Unit Delay/1  "Current"
  Saturation5/1 -> Vact/1
  Mux/1 -> Fcn2/1

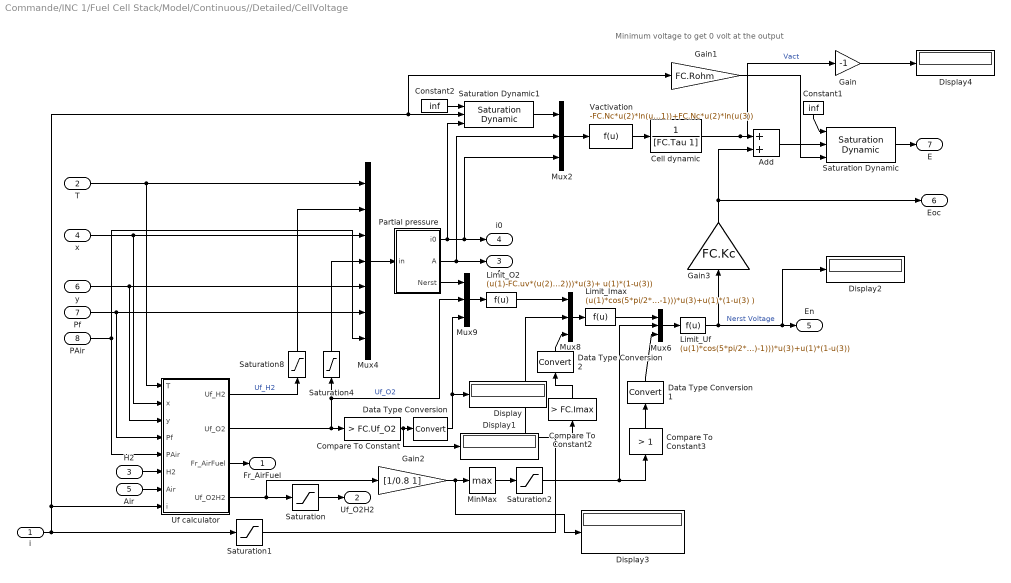
== system Commande/INC 1/Fuel Cell Stack/Model/Continuous//Detailed/CellVoltage ==
  note: Minimum voltage to get 0 volt at the output
  i : Inport
  T : Inport  Port=2
  H2 : Inport  Port=3
  x : Inport  Port=4
  Air : Inport  Port=5
  y : Inport  Port=6
  Pf : Inport  Port=7
  PAir : Inport  Port=8
  Add : Sum
  Cell dynamic : TransferFcn  Denominator=[FC.Tau 1]
  Compare To Constant : simulink/Logic and Bit Operations/Compare To Constant  relop=>  const=FC.Uf_O2  OutDataTypeStr=boolean
  Compare To Constant2 : simulink/Logic and Bit Operations/Compare To Constant  relop=>  const=FC.Imax  OutDataTypeStr=boolean
  Compare To Constant3 : simulink/Logic and Bit Operations/Compare To Constant  relop=>  const=1  OutDataTypeStr=boolean
  Constant1 : Constant  Value=inf
  Constant2 : Constant  Value=inf
  Data Type Conversion : DataTypeConversion
  Data Type Conversion1 : DataTypeConversion
  Data Type Conversion2 : DataTypeConversion
  Display{,1..4} (5 alike) : Display
  Gain : Gain  Gain=-1
  Gain1 : Gain  Gain=FC.Rohm
  Gain2 : Gain  Gain=[1/0.8 1]
  Gain3 : Gain  Gain=FC.Kc
  Limit_Imax : Fcn  Expr=(u(1)*cos(5*pi/2*(u(2)/FC.Imax-1)))*u(3)+u(1)*(1-u(3) )
  Limit_O2 : Fcn  Expr=(u(1)-FC.uv*(u(2)-FC.Uf_O2)/(FC.Kc*(FC.ufO2max-FC.Uf_O2)))*u(3)+ u(1)*(1-u(3))
  Limit_Uf : Fcn  Expr=(u(1)*cos(5*pi/2*(u(2)-1)))*u(3)+u(1)*(1-u(3))
  MinMax : MinMax  Function=max
  Mux{2,6,8..9} (4 alike) : Mux  Inputs=3
  Mux4 : Mux  Inputs=7
  Partial pressure : Subsystem
  Saturation : Saturate  UpperLimit=0.9999  LowerLimit=0.0001
  Saturation Dynamic : simulink/Discontinuities/Saturation Dynamic  OutMin=[]  OutMax=[]  OutDataTypeStr=Inherit: Same as second input  OutDataType=fixdt(1, 16)  OutScaling=2^-10  DoSatur=off
  Saturation Dynamic1 : simulink/Discontinuities/Saturation Dynamic  OutMin=[]  OutMax=[]  OutDataTypeStr=Inherit: Same as second input  OutDataType=fixdt(1, 16)  OutScaling=2^-10  DoSatur=off
  Saturation1 : Saturate  UpperLimit=FC.Imax*1.2  LowerLimit=0
  Saturation2 : Saturate  UpperLimit=1.2  LowerLimit=0
  Saturation4 : Saturate  UpperLimit=FC.Uf_O2  LowerLimit=0
  Saturation8 : Saturate  UpperLimit=FC.Uf_H2  LowerLimit=0
  Uf calculator : Subsystem
  Vactivation : Fcn  Expr=-FC.Nc*u(2)*ln(u(1))+FC.Nc*u(2)*ln(u(3))
  Fr_AirFuel : Outport  VectorParamsAs1DForOutWhenUnconnected=off
  Uf_O2H2 : Outport  Port=2  VectorParamsAs1DForOutWhenUnconnected=off
  A : Outport  Port=3  VectorParamsAs1DForOutWhenUnconnected=off
  i0 : Outport  Port=4  VectorParamsAs1DForOutWhenUnconnected=off
  En : Outport  Port=5  VectorParamsAs1DForOutWhenUnconnected=off
  Eoc : Outport  Port=6  VectorParamsAs1DForOutWhenUnconnected=off
  E : Outport  Port=7  VectorParamsAs1DForOutWhenUnconnected=off
  wires:
  Gain3/1 -> Eoc/1, Add/2
  Data Type Conversion1/1 -> Mux6/3
  Compare To Constant3/1 -> Data Type Conversion1/1
  Saturation2/1 -> Mux6/2, Compare To Constant3/1
  Saturation1/1 -> Mux8/2, Compare To Constant2/1
  Compare To Constant2/1 -> Data Type Conversion2/1
  Data Type Conversion2/1 -> Mux8/3
  Compare To Constant/1 -> Display1/1, Data Type Conversion/1
  Gain2/1 -> Display3/1, MinMax/1
  Partial pressure/3(Nerst) -> Mux9/1
  Saturation4/1 -> Mux4/4
  MinMax/1 -> Saturation2/1
  Saturation/1 -> Uf_O2H2/1
  Mux6/1 -> Limit_Uf/1
  Gain1/1 -> Saturation Dynamic/3
  Constant1/1 -> Saturation Dynamic/1
  Saturation Dynamic/1 -> E/1
  Add/1 -> Saturation Dynamic/2
  Cell dynamic/1 -> Gain/1, Add/1  "Vact"
  Vactivation/1 -> Cell dynamic/1
  Mux2/1 -> Vactivation/1
  Saturation Dynamic1/1 -> Mux2/1
  Constant2/1 -> Saturation Dynamic1/1
  Mux4/1 -> Partial pressure/1(in)
  Uf calculator/4(Uf_O2H2) -> Gain2/1, Saturation/1
  Saturation8/1 -> Mux4/2
  Limit_O2/1 -> Mux8/1
  Mux9/1 -> Limit_O2/1
  Uf calculator/3(Fr_AirFuel) -> Fr_AirFuel/1
  Limit_Uf/1 -> Gain3/1, Display2/1, En/1  "Nerst Voltage"
  Limit_Imax/1 -> Mux6/1
  Mux8/1 -> Limit_Imax/1
  Air/1 -> Uf calculator/7(Air)
  Uf calculator/2(Uf_O2) -> Mux9/2, Saturation4/1, Compare To Constant/1  "Uf_O2"
  Uf calculator/1(Uf_H2) -> Saturation8/1  "Uf_H2"
  i/1 -> Saturation1/1, Uf calculator/8(i), Gain1/1, Saturation Dynamic1/2
  H2/1 -> Uf calculator/6(H2)
  Partial pressure/2(A) -> Mux2/2, A/1
  Partial pressure/1(i0) -> Mux2/3, i0/1, Saturation Dynamic1/3
  PAir/1 -> Uf calculator/5(PAir), Mux4/7
  Pf/1 -> Uf calculator/4(Pf), Mux4/6
  y/1 -> Uf calculator/3(y), Mux4/5
  x/1 -> Uf calculator/2(x), Mux4/3
  T/1 -> Uf calculator/1(T), Mux4/1
  Data Type Conversion/1 -> Display/1, Mux9/3
  Gain/1 -> Display4/1

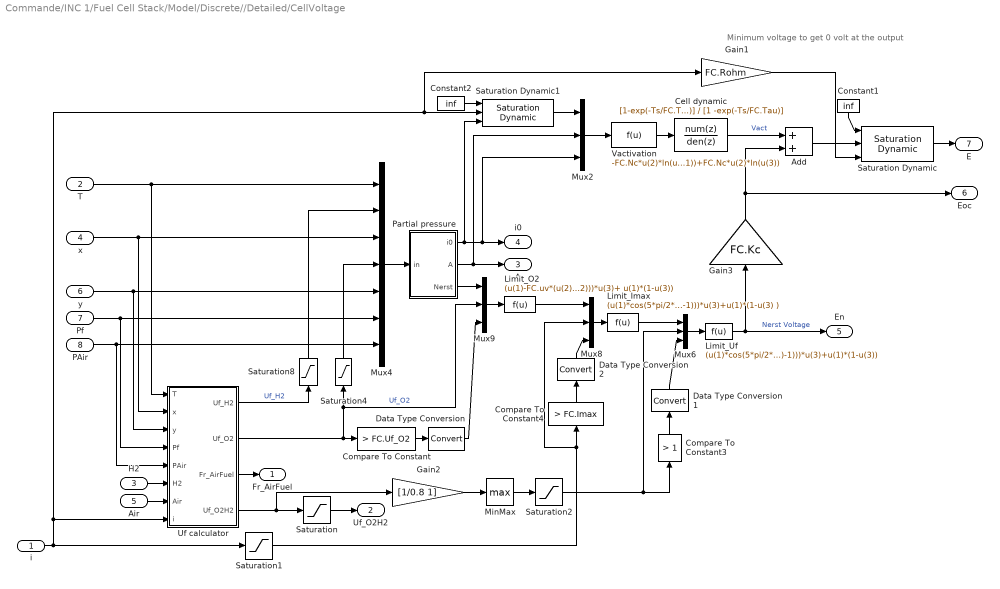
== system Commande/INC 1/Fuel Cell Stack/Model/Discrete//Detailed/CellVoltage ==
  note: Minimum voltage to get 0 volt at the output
  i : Inport
  T : Inport  Port=2
  H2 : Inport  Port=3
  x : Inport  Port=4
  Air : Inport  Port=5
  y : Inport  Port=6
  Pf : Inport  Port=7
  PAir : Inport  Port=8
  Add : Sum
  Cell dynamic : DiscreteTransferFcn  Numerator=[1-exp(-Ts/FC.Tau)]  Denominator=[1 -exp(-Ts/FC.Tau)]  SampleTime=Ts
  Compare To Constant : simulink/Logic and Bit Operations/Compare To Constant  relop=>  const=FC.Uf_O2  OutDataTypeStr=boolean
  Compare To Constant3 : simulink/Logic and Bit Operations/Compare To Constant  relop=>  const=1  OutDataTypeStr=boolean
  Compare To Constant4 : simulink/Logic and Bit Operations/Compare To Constant  relop=>  const=FC.Imax  OutDataTypeStr=boolean
  Constant1 : Constant  Value=inf
  Constant2 : Constant  Value=inf
  Data Type Conversion : DataTypeConversion
  Data Type Conversion1 : DataTypeConversion
  Data Type Conversion2 : DataTypeConversion
  Gain1 : Gain  Gain=FC.Rohm
  Gain2 : Gain  Gain=[1/0.8 1]
  Gain3 : Gain  Gain=FC.Kc
  Limit_Imax : Fcn  Expr=(u(1)*cos(5*pi/2*(u(2)/FC.Imax-1)))*u(3)+u(1)*(1-u(3) )
  Limit_O2 : Fcn  Expr=(u(1)-FC.uv*(u(2)-FC.Uf_O2)/(FC.Kc*(FC.ufO2max-FC.Uf_O2)))*u(3)+ u(1)*(1-u(3))
  Limit_Uf : Fcn  Expr=(u(1)*cos(5*pi/2*(u(2)-1)))*u(3)+u(1)*(1-u(3))
  MinMax : MinMax  Function=max
  Mux{2,6,8..9} (4 alike) : Mux  Inputs=3
  Mux4 : Mux  Inputs=7
  Partial pressure : Subsystem
  Saturation : Saturate  UpperLimit=0.9999  LowerLimit=0.0001
  Saturation Dynamic : simulink/Discontinuities/Saturation Dynamic  OutMin=[]  OutMax=[]  OutDataTypeStr=Inherit: Same as second input  OutDataType=fixdt(1, 16)  OutScaling=2^-10  DoSatur=off
  Saturation Dynamic1 : simulink/Discontinuities/Saturation Dynamic  OutMin=[]  OutMax=[]  OutDataTypeStr=Inherit: Same as second input  OutDataType=fixdt(1, 16)  OutScaling=2^-10  DoSatur=off
  Saturation1 : Saturate  UpperLimit=FC.Imax*1.2  LowerLimit=0
  Saturation2 : Saturate  UpperLimit=1.2  LowerLimit=0
  Saturation4 : Saturate  UpperLimit=FC.Uf_O2  LowerLimit=0
  Saturation8 : Saturate  UpperLimit=FC.Uf_H2  LowerLimit=0
  Uf calculator : Subsystem
  Vactivation : Fcn  Expr=-FC.Nc*u(2)*ln(u(1))+FC.Nc*u(2)*ln(u(3))
  Fr_AirFuel : Outport  VectorParamsAs1DForOutWhenUnconnected=off
  Uf_O2H2 : Outport  Port=2  VectorParamsAs1DForOutWhenUnconnected=off
  A : Outport  Port=3  VectorParamsAs1DForOutWhenUnconnected=off
  i0 : Outport  Port=4  VectorParamsAs1DForOutWhenUnconnected=off
  En : Outport  Port=5  VectorParamsAs1DForOutWhenUnconnected=off
  Eoc : Outport  Port=6  VectorParamsAs1DForOutWhenUnconnected=off
  E : Outport  Port=7  VectorParamsAs1DForOutWhenUnconnected=off
  wires:
  Gain3/1 -> Eoc/1, Add/2
  T/1 -> Uf calculator/1(T), Mux4/1
  x/1 -> Mux4/3, Uf calculator/2(x)
  y/1 -> Mux4/5, Uf calculator/3(y)
  Pf/1 -> Mux4/6, Uf calculator/4(Pf)
  PAir/1 -> Mux4/7, Uf calculator/5(PAir)
  Partial pressure/1(i0) -> Saturation Dynamic1/3, i0/1, Mux2/3
  Partial pressure/2(A) -> A/1, Mux2/2
  H2/1 -> Uf calculator/6(H2)
  i/1 -> Uf calculator/8(i), Saturation Dynamic1/2, Gain1/1, Saturation1/1
  Uf calculator/1(Uf_H2) -> Saturation8/1  "Uf_H2"
  Uf calculator/2(Uf_O2) -> Compare To Constant/1, Saturation4/1, Mux9/2  "Uf_O2"
  Air/1 -> Uf calculator/7(Air)
  Mux8/1 -> Limit_Imax/1
  Limit_Imax/1 -> Mux6/1
  Limit_Uf/1 -> Gain3/1, En/1  "Nerst Voltage"
  Uf calculator/3(Fr_AirFuel) -> Fr_AirFuel/1
  Mux9/1 -> Limit_O2/1
  Limit_O2/1 -> Mux8/1
  Saturation8/1 -> Mux4/2
  Uf calculator/4(Uf_O2H2) -> Saturation/1, Gain2/1
  Mux4/1 -> Partial pressure/1(in)
  Constant2/1 -> Saturation Dynamic1/1
  Saturation Dynamic1/1 -> Mux2/1
  Mux2/1 -> Vactivation/1
  Vactivation/1 -> Cell dynamic/1
  Cell dynamic/1 -> Add/1  "Vact"
  Add/1 -> Saturation Dynamic/2
  Saturation Dynamic/1 -> E/1
  Constant1/1 -> Saturation Dynamic/1
  Gain1/1 -> Saturation Dynamic/3
  Mux6/1 -> Limit_Uf/1
  Saturation/1 -> Uf_O2H2/1
  MinMax/1 -> Saturation2/1
  Saturation4/1 -> Mux4/4
  Partial pressure/3(Nerst) -> Mux9/1
  Gain2/1 -> MinMax/1
  Compare To Constant/1 -> Data Type Conversion/1
  Data Type Conversion/1 -> Mux9/3
  Data Type Conversion2/1 -> Mux8/3
  Compare To Constant4/1 -> Data Type Conversion2/1
  Saturation1/1 -> Mux8/2, Compare To Constant4/1
  Saturation2/1 -> Mux6/2, Compare To Constant3/1
  Compare To Constant3/1 -> Data Type Conversion1/1
  Data Type Conversion1/1 -> Mux6/3

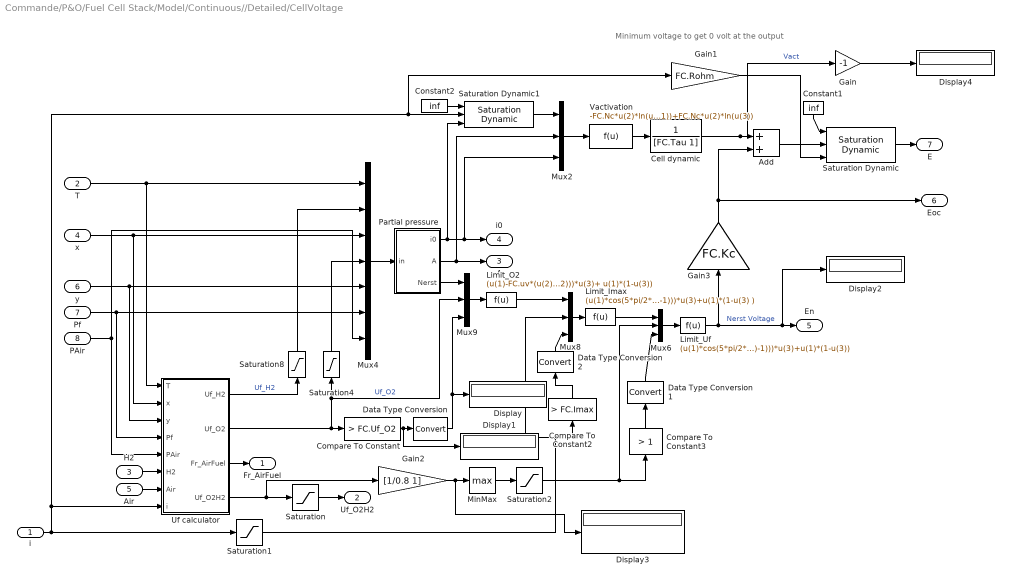
== system Commande/P&O/Fuel Cell Stack/Model/Continuous//Detailed/CellVoltage ==
  note: Minimum voltage to get 0 volt at the output
  i : Inport
  T : Inport  Port=2
  H2 : Inport  Port=3
  x : Inport  Port=4
  Air : Inport  Port=5
  y : Inport  Port=6
  Pf : Inport  Port=7
  PAir : Inport  Port=8
  Add : Sum
  Cell dynamic : TransferFcn  Denominator=[FC.Tau 1]
  Compare To Constant : simulink/Logic and Bit Operations/Compare To Constant  relop=>  const=FC.Uf_O2  OutDataTypeStr=boolean
  Compare To Constant2 : simulink/Logic and Bit Operations/Compare To Constant  relop=>  const=FC.Imax  OutDataTypeStr=boolean
  Compare To Constant3 : simulink/Logic and Bit Operations/Compare To Constant  relop=>  const=1  OutDataTypeStr=boolean
  Constant1 : Constant  Value=inf
  Constant2 : Constant  Value=inf
  Data Type Conversion : DataTypeConversion
  Data Type Conversion1 : DataTypeConversion
  Data Type Conversion2 : DataTypeConversion
  Display{,1..4} (5 alike) : Display
  Gain : Gain  Gain=-1
  Gain1 : Gain  Gain=FC.Rohm
  Gain2 : Gain  Gain=[1/0.8 1]
  Gain3 : Gain  Gain=FC.Kc
  Limit_Imax : Fcn  Expr=(u(1)*cos(5*pi/2*(u(2)/FC.Imax-1)))*u(3)+u(1)*(1-u(3) )
  Limit_O2 : Fcn  Expr=(u(1)-FC.uv*(u(2)-FC.Uf_O2)/(FC.Kc*(FC.ufO2max-FC.Uf_O2)))*u(3)+ u(1)*(1-u(3))
  Limit_Uf : Fcn  Expr=(u(1)*cos(5*pi/2*(u(2)-1)))*u(3)+u(1)*(1-u(3))
  MinMax : MinMax  Function=max
  Mux{2,6,8..9} (4 alike) : Mux  Inputs=3
  Mux4 : Mux  Inputs=7
  Partial pressure : Subsystem
  Saturation : Saturate  UpperLimit=0.9999  LowerLimit=0.0001
  Saturation Dynamic : simulink/Discontinuities/Saturation Dynamic  OutMin=[]  OutMax=[]  OutDataTypeStr=Inherit: Same as second input  OutDataType=fixdt(1, 16)  OutScaling=2^-10  DoSatur=off
  Saturation Dynamic1 : simulink/Discontinuities/Saturation Dynamic  OutMin=[]  OutMax=[]  OutDataTypeStr=Inherit: Same as second input  OutDataType=fixdt(1, 16)  OutScaling=2^-10  DoSatur=off
  Saturation1 : Saturate  UpperLimit=FC.Imax*1.2  LowerLimit=0
  Saturation2 : Saturate  UpperLimit=1.2  LowerLimit=0
  Saturation4 : Saturate  UpperLimit=FC.Uf_O2  LowerLimit=0
  Saturation8 : Saturate  UpperLimit=FC.Uf_H2  LowerLimit=0
  Uf calculator : Subsystem
  Vactivation : Fcn  Expr=-FC.Nc*u(2)*ln(u(1))+FC.Nc*u(2)*ln(u(3))
  Fr_AirFuel : Outport  VectorParamsAs1DForOutWhenUnconnected=off
  Uf_O2H2 : Outport  Port=2  VectorParamsAs1DForOutWhenUnconnected=off
  A : Outport  Port=3  VectorParamsAs1DForOutWhenUnconnected=off
  i0 : Outport  Port=4  VectorParamsAs1DForOutWhenUnconnected=off
  En : Outport  Port=5  VectorParamsAs1DForOutWhenUnconnected=off
  Eoc : Outport  Port=6  VectorParamsAs1DForOutWhenUnconnected=off
  E : Outport  Port=7  VectorParamsAs1DForOutWhenUnconnected=off
  wires:
  Gain3/1 -> Eoc/1, Add/2
  Data Type Conversion1/1 -> Mux6/3
  Compare To Constant3/1 -> Data Type Conversion1/1
  Saturation2/1 -> Mux6/2, Compare To Constant3/1
  Saturation1/1 -> Mux8/2, Compare To Constant2/1
  Compare To Constant2/1 -> Data Type Conversion2/1
  Data Type Conversion2/1 -> Mux8/3
  Compare To Constant/1 -> Display1/1, Data Type Conversion/1
  Gain2/1 -> Display3/1, MinMax/1
  Partial pressure/3(Nerst) -> Mux9/1
  Saturation4/1 -> Mux4/4
  MinMax/1 -> Saturation2/1
  Saturation/1 -> Uf_O2H2/1
  Mux6/1 -> Limit_Uf/1
  Gain1/1 -> Saturation Dynamic/3
  Constant1/1 -> Saturation Dynamic/1
  Saturation Dynamic/1 -> E/1
  Add/1 -> Saturation Dynamic/2
  Cell dynamic/1 -> Gain/1, Add/1  "Vact"
  Vactivation/1 -> Cell dynamic/1
  Mux2/1 -> Vactivation/1
  Saturation Dynamic1/1 -> Mux2/1
  Constant2/1 -> Saturation Dynamic1/1
  Mux4/1 -> Partial pressure/1(in)
  Uf calculator/4(Uf_O2H2) -> Gain2/1, Saturation/1
  Saturation8/1 -> Mux4/2
  Limit_O2/1 -> Mux8/1
  Mux9/1 -> Limit_O2/1
  Uf calculator/3(Fr_AirFuel) -> Fr_AirFuel/1
  Limit_Uf/1 -> Gain3/1, Display2/1, En/1  "Nerst Voltage"
  Limit_Imax/1 -> Mux6/1
  Mux8/1 -> Limit_Imax/1
  Air/1 -> Uf calculator/7(Air)
  Uf calculator/2(Uf_O2) -> Mux9/2, Saturation4/1, Compare To Constant/1  "Uf_O2"
  Uf calculator/1(Uf_H2) -> Saturation8/1  "Uf_H2"
  i/1 -> Saturation1/1, Uf calculator/8(i), Gain1/1, Saturation Dynamic1/2
  H2/1 -> Uf calculator/6(H2)
  Partial pressure/2(A) -> Mux2/2, A/1
  Partial pressure/1(i0) -> Mux2/3, i0/1, Saturation Dynamic1/3
  PAir/1 -> Uf calculator/5(PAir), Mux4/7
  Pf/1 -> Uf calculator/4(Pf), Mux4/6
  y/1 -> Uf calculator/3(y), Mux4/5
  x/1 -> Uf calculator/2(x), Mux4/3
  T/1 -> Uf calculator/1(T), Mux4/1
  Data Type Conversion/1 -> Display/1, Mux9/3
  Gain/1 -> Display4/1
